simulink model "clik_z_inverse"  (R2022b)
settings: Solver=ode1  StartTime=0.0  StopTime=4  FixedStep=0.001  RelTol=1e-3
undefined symbols (not defined in the file or in its folder): DiscIntNeverNeededParam, q0, Tc
settings Model: Creator=Xp  LastModifiedBy=shubham
settings SolverCC: AlgebraicLoopSolver=TrustRegion
settings DataIOCC: LimitDataPoints=on  SaveFormat=Array  SignalLoggingSaveFormat=ModelDataLogs  ReturnWorkspaceOutputs=off
settings OptimizationCC: ExpressionDepthLimit=2147483647  InitFltsAndDblsToZero=on  LifeSpan=inf
settings DebuggingCC: SaveWithParameterizedLinksMsg=none  UnderspecifiedInitializationDetection=Classic  MergeDetectMultiDrivingBlocksExec=none  SolverPrmCheckMsg=warning  MultiTaskDSMMsg=warning  MultiTaskCondExecSysMsg=none  FcnCallInpInsideContextMsg=warning  UnconnectedInputMsg=warning  UnconnectedOutputMsg=warning  UnconnectedLineMsg=warning  StateNameClashWarn=warning  SFUnexpectedBacktrackingDiag=warning  SFNoUnconditionalDefaultTransitionDiag=warning  SFExecutionAtInitializationDiag=none  SFMachineParentedDataDiag=warning  ArithmeticOperatorsInVariantConditions=warning
settings HardwareCC: ProdBitPerPointer=32  ProdBitPerSizeT=32  ProdBitPerPtrDiffT=32  ProdLargestAtomicFloat=None  ProdIntDivRoundTo=Undefined  ProdEndianess=Unspecified  ProdWordSize=32  ProdHWDeviceType=32-bit Generic
settings ModelReferenceCC: EnableRefExpFcnMdlSchedulingChecks=on  PropagateSignalLabelsOutOfModel=off
settings SFSimCC: CustomCodeUndefinedFunction=UseInterfaceOnly
settings RTWCC: DLArmComputeVersion=19.05
settings CodeAppCC: StateflowObjectComments=on
settings GRTTargetCC: TargetLangStandard=C89/C90 (ANSI)  CombineOutputUpdateFcns=off  GRTInterface=on
settings ConfigComp: CovMetricSettings=dw  CovSaveCumulativeToWorkspaceVar=on  CovSaveSingleToWorkspaceVar=on

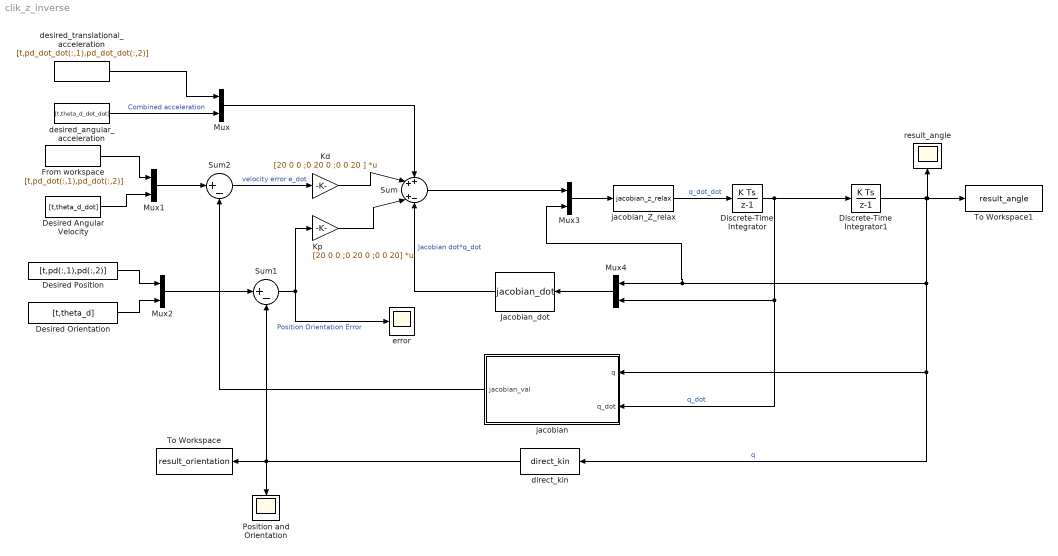
== system clik_z_inverse ==
  Desired Angular Velocity : FromWorkspace  VariableName=[t,theta_d_dot]
  Desired Orientation : FromWorkspace  VariableName=[t,theta_d]
  Desired Position : FromWorkspace  VariableName=[t,pd(:,1),pd(:,2)]
  Discrete-Time Integrator : DiscreteIntegrator  InitialCondition=[0;0;0;0]  SampleTime=Tc  ICPrevOutput=DiscIntNeverNeededParam  ICPrevScaledInput=DiscIntNeverNeededParam
  Discrete-Time Integrator1 : DiscreteIntegrator  InitialCondition=q0  SampleTime=Tc  LimitOutput=on  UpperSaturationLimit=[inf;inf;1;inf]  LowerSaturationLimit=[-inf; -inf; 0.25; -inf]  ICPrevOutput=DiscIntNeverNeededParam  ICPrevScaledInput=DiscIntNeverNeededParam
  From workspace : FromWorkspace  VariableName=[t,pd_dot(:,1),pd_dot(:,2)]
  Jacobian_dot : MATLABFcn  MATLABFcn=jacobian_dot  OutputDimensions=3
  Kd : Gain  Gain=[20 0 0 ;0 20 0 ;0 0 20 ]  Multiplication=Matrix(K*u)
  Kp : Gain  Gain=[20 0 0 ;0 20 0 ;0 0 20]  Multiplication=Matrix(K*u)
  Mux{,1..4} (5 alike) : Mux  Inputs=2
  Position and Orientation : Scope
  Sum : Sum  Inputs=++|+-
  Sum1 : Sum  Inputs=|+-
  Sum2 : Sum  Inputs=|+-
  To Workspace : ToWorkspace  VariableName=result_orientation  SampleTime=-1
  To Workspace1 : ToWorkspace  VariableName=result_angle  SampleTime=-1
      settings: Save2DSignal=2-D array (concatenate along first dimension)
  desired_angular_acceleration : FromWorkspace  VariableName=[t,theta_d_dot_dot]
  "desired_translational_acceleration " : FromWorkspace  VariableName=[t,pd_dot_dot(:,1),pd_dot_dot(:,2)]
  direct_kin : MATLABFcn  MATLABFcn=direct_kin  OutputDimensions=3
  error : Scope
  "jacobian " : MATLAB Function  TreatAsAtomicUnit=on
  jacobian_Z_relax : MATLABFcn  MATLABFcn=jacobian_z_relax  OutputDimensions=4
  result_angle : Scope
  wires:
  Mux2/1 -> Sum1/1
  "jacobian "/1(jacobian_val) -> Sum2/2
  Sum2/1 -> Kd/1  "velocity error e_dot"
  direct_kin/1 -> Sum1/2, To Workspace/1, Position and Orientation/1
  Sum1/1 -> error/1, Kp/1  "Position Orientation Error"
  Discrete-Time Integrator/1 -> Mux4/2, "jacobian "/2(q_dot), Discrete-Time Integrator1/1  "q_dot"
  jacobian_Z_relax/1 -> Discrete-Time Integrator/1  "q_dot_dot"
  Discrete-Time Integrator1/1 -> Mux3/2, Mux4/1, "jacobian "/1(q), direct_kin/1, To Workspace1/1, result_angle/1  "q"
  Mux4/1 -> Jacobian_dot/1
  Kd/1 -> Sum/2
  Kp/1 -> Sum/3
  Mux3/1 -> jacobian_Z_relax/1
  Jacobian_dot/1 -> Sum/4  "Jacobian dot*q_dot"
  Mux/1 -> Sum/1
  "desired_translational_acceleration "/1 -> Mux/1
  desired_angular_acceleration/1 -> Mux/2  "Combined acceleration"
  From workspace/1 -> Mux1/1
  Mux1/1 -> Sum2/1
  Desired Angular Velocity/1 -> Mux1/2
  Desired Position/1 -> Mux2/1
  Desired Orientation/1 -> Mux2/2
  Sum/1 -> Mux3/1

== matlab function clik_z_inverse/jacobian  ==
  data: q input; jacobian_val output; q_dot input
function jacobian_val= fcn(q,q_dot)
    %input parameters
    theta1=q(1);
    theta2=q(2);
    
    %robot parameters
    a1 = 0.5;
    a2 = 0.5;
    
    jacobian_mat=[-a2*sin(theta1 + theta2) - a1*sin(theta1), -a2*sin(theta1 + theta2), 0, 0;
        a2*cos(theta1 + theta2) + a1*cos(theta1), a2*cos(theta1 + theta2), 0, 0;
        1, 1, 0, 1];
    
    jacobian_val=jacobian_mat*q_dot;

end
